simulink model "Junctions2"  (Simulink 9.0)
settings: Solver=FixedStepDiscrete  StartTime=0.0  StopTime=10.0  RelTol=1e-3  EnableMultiTasking=on
model workspace (MAT data in the model file):
  x3 = Simulink.Parameter
  x3.Value = 333
  x3.DataType = 'int32'
  x3.Dimensions = [1 1]
  x4 = Simulink.Parameter
  x4.Value = 542
  x4.DataType = 'double'
  x4.Dimensions = [1 1]
settings Model: SuppressorTable=22 serialization::archive 11 0 6 0 0 0 0 0  Creator=scaife  LastModifiedBy=hbourbou  ExtModeAutoUpdateStatusClock=off
settings DataIOCC: LimitDataPoints=on  SignalLoggingSaveFormat=ModelDataLogs  SignalLoggingName=sigsOut
settings DebuggingCC: SaveWithParameterizedLinksMsg=none  SignalResolutionControl=TryResolveAllWithWarning  MultiTaskDSMMsg=warning  MultiTaskCondExecSysMsg=none
settings HardwareCC: TargetUnknown=on
settings SFSimCC: SimParseCustomCode=off
settings GRTTargetCC: GeneratePreprocessorConditionals=Disable all  CombineOutputUpdateFcns=off  GRTInterface=on

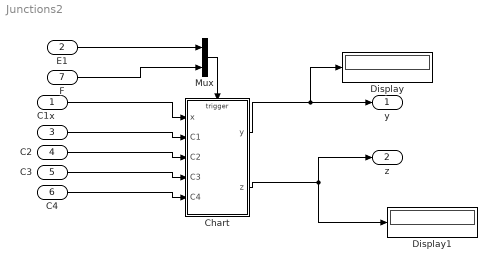
== system Junctions2 ==
  x : Inport
  E1 : Inport  Port=2
  C1 : Inport  Port=3
  C2 : Inport  Port=4
  C3 : Inport  Port=5
  C4 : Inport  Port=6
  F : Inport  Port=7
  Chart : Stateflow chart  TreatAsAtomicUnit=on
  Display : Display
  Display1 : Display
  Mux : Mux  Inputs=2
  y : Outport
  z : Outport  Port=2
  wires:
  x/1 -> Chart/1(x)
  E1/1 -> Mux/1
  Chart/1(y) -> Display/1, y/1
  Chart/2(z) -> z/1, Display1/1
  C1/1 -> Chart/2(C1)
  C2/1 -> Chart/3(C2)
  C3/1 -> Chart/4(C3)
  C4/1 -> Chart/5(C4)
  Mux/1 -> Chart/Trigger
  F/1 -> Mux/2

== stateflow chart Chart ==
  state A
    en: y = 0;
    x1 = 0;
    z = 0;
    ex : y=2.*x3+x4
  state C
    du : x1 = x1 + 1;
  state B
    du : x1 = x1 - 1;
  state D
    du : x1 = x1 + 1;
  (junction 21) -> (junction 20) [order 3]
  A -> (junction 21) [order 1] : E1[C1]{y = y + 1;z=2+x2}
  (junction 21) -> B [order 1] : F[C2]{y=2;x1 = x1 + 1}
  (default) -> A
  (junction 21) -> D [order 2] : [C3]
  A -> C [order 2] : [C4]{y = y + 1;z = z + 1}
  data: x input double; y output double =1; z output double =2; C1 input boolean; C2 input boolean; C3 input boolean; C4 input boolean; x1 local double; x2 constant double; x3 parameter double; x4 parameter double
  events: E1 input FALLING_EDGE_EVENT; F input RISING_EDGE_EVENT
